simulink model "fsk_block_implementation"  (R2021a)
settings: Solver=VariableStepAuto  StartTime=0.0  StopTime=10  RelTol=1e-3
libraries: commchan3 x3, commsink2 x3, commdigbbndpm3 x2, commdigbbndfm2 x2, commdigbbndam3 x2, commrandsrc3 x2, dspsrcs4 x1, dspquant2 x1
settings Model: Creator=Yash  LastModifiedBy=Yash

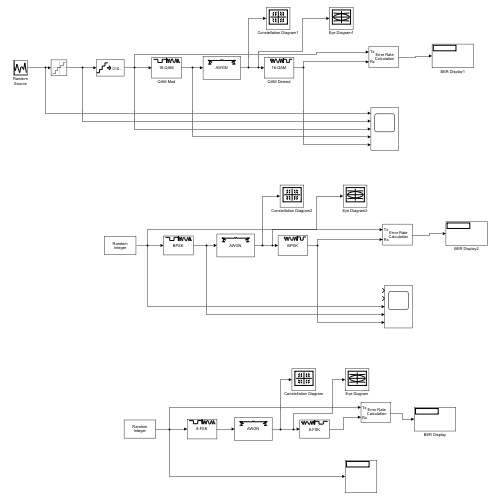
[thumbnail: Simulink's stored preview of the top-level diagram]
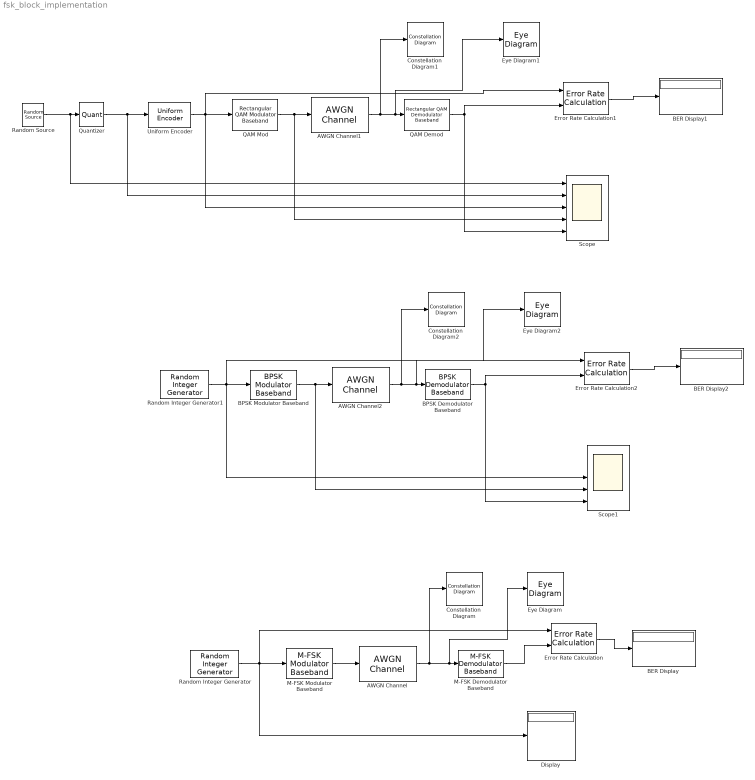
== system fsk_block_implementation ==
  AWGN Channel : commchan3/AWGN Channel  InputProcessing=Columns as channels (frame based)  seed=67  noiseMode="Signal to noise ratio  (Eb/No)"  EbNodB=-10  EsNodB=10  SNRdB=10  bitsPerSym=1  Ps=1  Tsym=1  variance=1
  AWGN Channel1 : commchan3/AWGN Channel  InputProcessing=Columns as channels (frame based)  seed=67  noiseMode="Signal to noise ratio  (Eb/No)"  EbNodB=-10  EsNodB=10  SNRdB=10  bitsPerSym=1  Ps=1  Tsym=1  variance=1
  AWGN Channel2 : commchan3/AWGN Channel  InputProcessing=Columns as channels (frame based)  seed=67  noiseMode="Signal to noise ratio  (Eb/No)"  EbNodB=-10  EsNodB=10  SNRdB=10  bitsPerSym=1  Ps=1  Tsym=1  variance=1
  BER Display : Display
  BER Display1 : Display
  BER Display2 : Display
  BPSK Demodulator Baseband : commdigbbndpm3/BPSK Demodulator Baseband  DecType=Hard decision  VarSource=Dialog  Variance=1  Ph=0  outDtype=Inherit via internal rule  derotateFactorWordLen=16  derotateFactorDataTypeStr=Inherit: Same word length as input  derotateFactorLastDataTypeStr=Inherit: Same word length as input
  BPSK Modulator Baseband : commdigbbndpm3/BPSK Modulator Baseband  Ph=0  outDtype=double  outWordLen=16  outUDDataType=sfix(16)  outFracLenMode=Best precision  outFracLen=15  outDataTypeStr=double  outLastDataTypeStr=double
  Constellation Diagram : ConstellationDiagram
  Constellation Diagram1 : ConstellationDiagram
  Constellation Diagram2 : ConstellationDiagram
  Display : Display
  Error Rate Calculation : commsink2/Error Rate Calculation  N=0  st_delay=0  cp_mode=Entire frame  subframe=[]  PMode=Port  WsName=ErrorVec  RsMode2=off  stop=off  numErr=100  maxBits=1e6
  Error Rate Calculation1 : commsink2/Error Rate Calculation  N=0  st_delay=0  cp_mode=Entire frame  subframe=[]  PMode=Port  WsName=ErrorVec  RsMode2=off  stop=off  numErr=100  maxBits=1e6
  Error Rate Calculation2 : commsink2/Error Rate Calculation  N=0  st_delay=0  cp_mode=Entire frame  subframe=[]  PMode=Port  WsName=ErrorVec  RsMode2=off  stop=off  numErr=100  maxBits=1e6
  Eye Diagram : EyeDiagram
  Eye Diagram1 : EyeDiagram
  Eye Diagram2 : EyeDiagram
  M-FSK Demodulator Baseband : commdigbbndfm2/M-FSK Demodulator Baseband  M=8  OutType=Integer  Dec=Gray  freqSep=6  numSamp=17  RateOptions=Enforce single-rate processing  outDataType=double
      settings: SourceProductBaseCode=CM
  M-FSK Modulator Baseband : commdigbbndfm2/M-FSK Modulator Baseband  M=8  InType=Integer  Enc=Gray  freqSep=6  phaseType=Continuous  numSamp=17  RateOptions=Enforce single-rate processing  outDataType=double
  QAM Demod : commdigbbndam3/Rectangular QAM Demodulator Baseband  M=16  OutType=Integer  DecType=Hard decision  VarSource=Dialog  Variance=1  Dec=Gray  Mapping=[0:15]  PowType=Min. distance between symbols  MinDist=2  AvgPow=1  PeakPow=1  Ph=0  outDtype1=Inherit via internal rule  outDtype2=Inherit via internal rule  derotateFactorWordLen=16  derotateFactorDataTypeStr=Inherit: Same word length as input  derotateFactorLastDataTypeStr=Inherit: Same word length as input  denormFactorWordLen=16  denormFactorDataTypeStr=Inherit: Same word length as input  denormFactorLastDataTypeStr=Inherit: Same word length as input  prodOutWordLen=32  prodOutOverflowMode=Wrap  prodOutRoundingMode=Floor  prodOutOvFlMode=off  prodOutOvFlModeLastStrValue=off  sumWordLen=32
  QAM Mod : commdigbbndam3/Rectangular QAM Modulator Baseband  M=16  InType=Integer  Enc=Gray  Mapping=[0:15]  PowType=Min. distance between symbols  MinDist=2  AvgPow=1  PeakPow=1  Ph=0  outDtype=double  outWordLen=16  outUDDataType=sfix(16)  outFracLenMode=Best precision  outFracLen=15  outDataTypeStr=double  outLastDataTypeStr=double
  Quantizer : Quantizer  QuantizationInterval=0.25  LinearizeAsGain=off
  Random Source : dspsrcs4/Random Source  SrcType=Uniform  NormMethod=Ziggurat  CltLength=12  MinVal=0  MaxVal=1  MeanVal=0  VarVal=1  RepMode=Not repeatable  rawSeed=1  IsInherit=off  SampMode=Discrete  SampTime=0.1  SampFrame=1  DataType=Single  OutComplex=Real  OutputFrames=off
  Random Integer Generator : commrandsrc3/Random Integer Generator  SetSize=8  SeedSource=Auto  Seed=0  SampleTime=1  SamplesPerFrame=100  OutputDataType=double  SimulateUsing=Interpreted execution
  Random Integer Generator1 : commrandsrc3/Random Integer Generator  SetSize=2  SeedSource=Auto  Seed=0  SampleTime=0.1  SamplesPerFrame=1  OutputDataType=double  SimulateUsing=Interpreted execution
  Scope : Scope  NumInputPorts=5
  Scope1 : Scope  NumInputPorts=5
  Uniform Encoder : dspquant2/Uniform Encoder  peak=1  bits=4  otype=Unsigned integer
  wires:
  Error Rate Calculation1/1 -> BER Display1/1
  QAM Mod/1 -> AWGN Channel1/1, Scope/4
  Quantizer/1 -> Uniform Encoder/1, Scope/2
  AWGN Channel1/1 -> Eye Diagram1/1, QAM Demod/1, Constellation Diagram1/1
  Uniform Encoder/1 -> QAM Mod/1, Error Rate Calculation1/1, Scope/3
  Random Source/1 -> Scope/1, Quantizer/1
  QAM Demod/1 -> Error Rate Calculation1/2, Scope/5
  Random Integer Generator1/1 -> BPSK Modulator Baseband/1, Error Rate Calculation2/1, Scope1/3
  AWGN Channel2/1 -> BPSK Demodulator Baseband/1, Eye Diagram2/1, Constellation Diagram2/1
  Error Rate Calculation2/1 -> BER Display2/1
  BPSK Demodulator Baseband/1 -> Error Rate Calculation2/2, Scope1/5
  BPSK Modulator Baseband/1 -> AWGN Channel2/1, Scope1/4
  AWGN Channel/1 -> Eye Diagram/1, M-FSK Demodulator Baseband/1, Constellation Diagram/1
  M-FSK Demodulator Baseband/1 -> Error Rate Calculation/2
  Error Rate Calculation/1 -> BER Display/1
  Random Integer Generator/1 -> Display/1, Error Rate Calculation/1, M-FSK Modulator Baseband/1
  M-FSK Modulator Baseband/1 -> AWGN Channel/1
